simulink library "GenericINSLibrary"  (R2020b)
settings: Solver=VariableStepAuto  StartTime=0.0  StopTime=10.0  RelTol=1e-3
libraries: simulink x44
(part 5 of 6)

== matlab function GenericINSLibrary/Sensor Fusion/MATLAB Function ==
  data: time input; initialState input; valid output; initialStdDev input; reset input; sampletime input; IMU_Data input; IMU_StdDev input; IMU_PositionBody2Sensor input; IMU_DCMBody2Sensor input; P1_Data input; P1_StdDev input; P1_PositionBody2Sensor input; P2_Data input; P2_StdDev input; P2_PositionBody2Sensor input; P3_Data input; P3_StdDev input; P3_PositionBody2Sensor input; P4_Data input; P4_StdDev input; P4_PositionBody2Sensor input; P5_Data input; P5_StdDev input; P5_PositionBody2Sensor input; P6_Data input; P6_StdDev input; P6_PositionBody2Sensor input; V1_Data input; V1_StdDev input; V1_PositionBody2Sensor input; V1_DCMBody2Sensor input; V2_Data input; V2_StdDev input; V2_PositionBody2Sensor input; V2_DCMBody2Sensor input; V3_Data input; V3_StdDev input; V3_PositionBody2Sensor input; V3_DCMBody2Sensor input; V4_Data input; V4_StdDev input; V4_PositionBody2Sensor input; V4_DCMBody2Sensor input; O1_Data input; O1_StdDev input; O1_DCMBody2Sensor input; O2_Data input; O2_StdDev input; O2_DCMBody2Sensor input; O3_Data input; O3_StdDev input; O3_DCMBody2Sensor input; O4_Data input; O4_StdDev input; O4_DCMBody2Sensor input; SOG1_Data input; SOG1_StdDev input; SOG1_PositionBody2Sensor input; SOG2_Data input; SOG2_StdDev input; SOG2_PositionBody2Sensor input; SOG3_Data input; SOG3_StdDev input; SOG3_PositionBody2Sensor input; SOG4_Data input; SOG4_StdDev input; SOG4_PositionBody2Sensor input; SOG5_Data input; SOG5_StdDev input; SOG5_PositionBody2Sensor input; SOG6_Data input; SOG6_StdDev input; SOG6_PositionBody2Sensor input; numPredictions output; numUpdates output; positionLLA output; orientationQuaternionWXYZ output; orientationRollPitchYaw output; velocityNED output; velocityUVW output; velocityPQR output; courseOverGround output; speedOverGround output; angleOfAttack output; sideSlipAngle output; inertialSensorBias output; internalX output; internalS output
function [valid, numPredictions, numUpdates, positionLLA, orientationQuaternionWXYZ, orientationRollPitchYaw, velocityNED, velocityUVW, velocityPQR, courseOverGround, speedOverGround, angleOfAttack, sideSlipAngle, inertialSensorBias, internalX, internalS] = MultiSensorFusion(time, initialState, initialStdDev, reset, sampletime, IMU_Data, IMU_StdDev, IMU_PositionBody2Sensor, IMU_DCMBody2Sensor, P1_Data, P1_StdDev, P1_PositionBody2Sensor, P2_Data, P2_StdDev, P2_PositionBody2Sensor, P3_Data, P3_StdDev, P3_PositionBody2Sensor, P4_Data, P4_StdDev, P4_PositionBody2Sensor, P5_Data, P5_StdDev, P5_PositionBody2Sensor, P6_Data, P6_StdDev, P6_PositionBody2Sensor, V1_Data, V1_StdDev, V1_PositionBody2Sensor, V1_DCMBody2Sensor, V2_Data, V2_StdDev, V2_PositionBody2Sensor, V2_DCMBody2Sensor, V3_Data, V3_StdDev, V3_PositionBody2Sensor, V3_DCMBody2Sensor, V4_Data, V4_StdDev, V4_PositionBody2Sensor, V4_DCMBody2Sensor, O1_Data, O1_StdDev, O1_DCMBody2Sensor, O2_Data, O2_StdDev, O2_DCMBody2Sensor, O3_Data, O3_StdDev, O3_DCMBody2Sensor, O4_Data, O4_StdDev, O4_DCMBody2Sensor, SOG1_Data, SOG1_StdDev, SOG1_PositionBody2Sensor, SOG2_Data, SOG2_StdDev, SOG2_PositionBody2Sensor, SOG3_Data, SOG3_StdDev, SOG3_PositionBody2Sensor, SOG4_Data, SOG4_StdDev, SOG4_PositionBody2Sensor, SOG5_Data, SOG5_StdDev, SOG5_PositionBody2Sensor, SOG6_Data, SOG6_StdDev, SOG6_PositionBody2Sensor)
    %MultiSensorFusion Generated MATLAB function for a generic inertial navigation system (6 position measurements, 4 velocity measurements, 4 orientation measurements).
    % This function was automatically generated using the command GenericINS.SensorFusion.GenerateFunction('MultiSensorFusion', [3  3  3  3  3  3], [3  3  2  2], [3  3  1  1], 6).
    % 
    % PARAMETERS
    % time                       ... A scalar value indicating a monotonically increasing time in seconds.
    % initialState               ... 15-by-1 initial state vector to be used when the INS is reset. The elements are as follows:
    %                                 1: latitude     [rad]     Initial latitude of the position of the IMU.
    %                                 2: longitude    [rad]     Initial longitude of the position of the IMU.
    %                                 3: altitude     [m]       Initial altitude of the position of the IMU, positive upwards.
    %                                 4: velocityU    [m/s]     Initial body-fixed velocity in x-direction of the body-frame at the position of the IMU.
    %                                 5: velocityV    [m/s]     Initial body-fixed velocity in y-direction of the body-frame at the position of the IMU.
    %                                 6: velocityW    [m/s]     Initial body-fixed velocity in z-direction of the body-frame at the position of the IMU.
    %                                 7: roll         [rad]     Initial roll angle.
    %                                 8: pitch        [rad]     Initial pitch angle.
    %                                 9: yaw          [rad]     Initial yaw angle.
    %                                10: biasAccX     [m/(s*s)] Initial acceleration bias in x-direction of IMU sensor frame.
    %                                11: biasAccY     [m/(s*s)] Initial acceleration bias in y-direction of IMU sensor frame.
    %                                12: biasAccZ     [m/(s*s)] Initial acceleration bias in z-direction of IMU sensor frame.
    %                                13: biasGyrX     [rad/s]   Initial angular rate bias around x-axis of IMU sensor frame.
    %                                14: biasGyrY     [rad/s]   Initial angular rate bias around y-axis of IMU sensor frame.
    %                                15: biasGyrZ     [rad/s]   Initial angular rate bias around z-axis of IMU sensor frame.
    % initialStdDev              ... 15-by-1 standard deviation vector that represents the unvertainty of the initial state. It is better to use larger values than
    %                                too small values for the filter to converge. The elements are as follows:
    %                                 1: latitude     [rad]     Initial standard deviation for initial latitude.
    %                                 2: longitude    [rad]     Initial standard deviation for initial longitude.
    %                                 3: altitude     [m]       Initial standard deviation for initial altitude.
    %                                 4: velocityU    [m/s]     Initial standard deviation for initial body-fixed velocity in x-direction of the body-frame.
    %                                 5: velocityV    [m/s]     Initial standard deviation for initial body-fixed velocity in y-direction of the body-frame.
    %                                 6: velocityW    [m/s]     Initial standard deviation for initial body-fixed velocity in z-direction of the body-frame.
    %                                 7: orientationX           Initial standard deviation for x-component of orientation vector (axis-angle representation).
    %                                 8: orientationY           Initial standard deviation for y-component of orientation vector (axis-angle representation).
    %                                 9: orientationZ           Initial standard deviation for z-component of orientation vector (axis-angle representation).
    %                                10: biasAccX     [m/(s*s)] Initial standard deviation for acceleration bias in x-direction of IMU sensor frame.
    %                                11: biasAccY     [m/(s*s)] Initial standard deviation for acceleration bias in y-direction of IMU sensor frame.
    %                                12: biasAccZ     [m/(s*s)] Initial standard deviation for acceleration bias in z-direction of IMU sensor frame.
    %                                13: biasGyrX     [rad/s]   Initial standard deviation for angular rate bias around x-axis of IMU sensor frame.
    %                                14: biasGyrY     [rad/s]   Initial standard deviation for angular rate bias around y-axis of IMU sensor frame.
    %                                15: biasGyrZ     [rad/s]   Initial standard deviation for angular rate bias around z-axis of IMU sensor frame.
    % reset                      ... Greater than 0.0 if filter should be reset/reinitialized, 0.0 otherwise. During an initialization the initial state and initial standard deviations are used.
    % sampletime                 ... Discrete sampletime in seconds to be used for forward euler integration. Should be the elapsed time to the latest prediction.
    % IMU_Data                   ... The 7-by-1 vector representing the IMU data where the elements are as follows:
    %                                 1: trigger                Greater than 0.0 if new IMU data is available and should be used in a prediction step, 0.0 otherwise.
    %                                 2: accX         [m/(s*s)] Acceleration in x-direction of IMU sensor frame.
    %                                 3: accY         [m/(s*s)] Acceleration in y-direction of IMU sensor frame.
    %                                 4: accZ         [m/(s*s)] Acceleration in z-direction of IMU sensor frame.
    %                                 5: gyrX         [rad/s]   Angular rate around x-axis of IMU sensor frame.
    %                                 6: gyrY         [rad/s]   Angular rate around y-axis of IMU sensor frame.
    %                                 7: gyrZ         [rad/s]   Angular rate around z-axis of IMU sensor frame.
    % IMU_StdDev                 ... 12-by-1 vector representing the standard deviation for inertial measurements and inertial biases. The elements are as follows:
    %                                 1: accX         [m/(s*s)] Standard deviation for acceleration in x-direction of IMU sensor frame.
    %                                 2: accY         [m/(s*s)] Standard deviation for acceleration in y-direction of IMU sensor frame.
    %                                 3: accZ         [m/(s*s)] Standard deviation for acceleration in z-direction of IMU sensor frame.
    %                                 4: gyrX         [rad/s]   Standard deviation for angular rate around x-axis of IMU sensor frame.
    %                                 5: gyrY         [rad/s]   Standard deviation for angular rate around y-axis of IMU sensor frame.
    %                                 6: gyrZ         [rad/s]   Standard deviation for angular rate around z-axis of IMU sensor frame.
    %                                 7: biasAccX     [m/(s*s)] Standard deviation for acceleration bias in x-direction of IMU sensor frame.
    %                                 8: biasAccY     [m/(s*s)] Standard deviation for acceleration bias in y-direction of IMU sensor frame.
    %                                 9: biasAccZ     [m/(s*s)] Standard deviation for acceleration bias in z-direction of IMU sensor frame.
    %                                10: biasGyrX     [rad/s]   Standard deviation for angular rate bias around x-axis of IMU sensor frame.
    %                                11: biasGyrY     [rad/s]   Standard deviation for angular rate bias around y-axis of IMU sensor frame.
    %                                12: biasGyrZ     [rad/s]   Standard deviation for angular rate bias around z-axis of IMU sensor frame.
    % IMU_PositionBody2Sensor    ... Position of IMU sensor frame origin w.r.t. body frame origin in body frame coordinates (meters).
    % IMU_DCMBody2Sensor         ... Direction cosine matrix to rotate measurements from body frame to sensor frame.
    % P1_Data                    ... 4-by-1 vector representing the position measurements of position sensor 1. The elements are as follows:
    %                                 1: trigger                Greater than 0.0 if new measurement data is available and should be used in an update step, 0.0 otherwise.
    %                                 2: latitude     [rad]     The latitude measurement.
    %                                 3: longitude    [rad]     The longitude measurement.
    %                                 4: altitude     [m]       The altitude measurement.
    % P1_StdDev                  ... 3-by-1 vector representing the standard deviation for the position measurements of position sensor 1. The elements are as follows:
    %                                 1: stdNorth     [m]       Standard deviation in north direction.
    %                                 2: stdEast      [m]       Standard deviation in east direction.
    %                                 3: stdDown      [m]       Standard deviation in up/down-direction.
    % P1_PositionBody2Sensor     ... Position of position sensor 1 w.r.t. body frame origin in body frame coordinates (meters).
    % P2_Data                    ... 4-by-1 vector representing the position measurements of position sensor 2. The elements are as follows:
    %                                 1: trigger                Greater than 0.0 if new measurement data is available and should be used in an update step, 0.0 otherwise.
    %                                 2: latitude     [rad]     The latitude measurement.
    %                                 3: longitude    [rad]     The longitude measurement.
    %                                 4: altitude     [m]       The altitude measurement.
    % P2_StdDev                  ... 3-by-1 vector representing the standard deviation for the position measurements of position sensor 2. The elements are as follows:
    %                                 1: stdNorth     [m]       Standard deviation in north direction.
    %                                 2: stdEast      [m]       Standard deviation in east direction.
    %                                 3: stdDown      [m]       Standard deviation in up/down-direction.
    % P2_PositionBody2Sensor     ... Position of position sensor 2 w.r.t. body frame origin in body frame coordinates (meters).
    % P3_Data                    ... 4-by-1 vector representing the position measurements of position sensor 3. The elements are as follows:
    %                                 1: trigger                Greater than 0.0 if new measurement data is available and should be used in an update step, 0.0 otherwise.
    %                                 2: latitude     [rad]     The latitude measurement.
    %                                 3: longitude    [rad]     The longitude measurement.
    %                                 4: altitude     [m]       The altitude measurement.
    % P3_StdDev                  ... 3-by-1 vector representing the standard deviation for the position measurements of position sensor 3. The elements are as follows:
    %                                 1: stdNorth     [m]       Standard deviation in north direction.
    %                                 2: stdEast      [m]       Standard deviation in east direction.
    %                                 3: stdDown      [m]       Standard deviation in up/down-direction.
    % P3_PositionBody2Sensor     ... Position of position sensor 3 w.r.t. body frame origin in body frame coordinates (meters).
    % P4_Data                    ... 4-by-1 vector representing the position measurements of position sensor 4. The elements are as follows:
    %                                 1: trigger                Greater than 0.0 if new measurement data is available and should be used in an update step, 0.0 otherwise.
    %                                 2: latitude     [rad]     The latitude measurement.
    %                                 3: longitude    [rad]     The longitude measurement.
    %                                 4: altitude     [m]       The altitude measurement.
    % P4_StdDev                  ... 3-by-1 vector representing the standard deviation for the position measurements of position sensor 4. The elements are as follows:
    %                                 1: stdNorth     [m]       Standard deviation in north direction.
    %                                 2: stdEast      [m]       Standard deviation in east direction.
    %                                 3: stdDown      [m]       Standard deviation in up/down-direction.
    % P4_PositionBody2Sensor     ... Position of position sensor 4 w.r.t. body frame origin in body frame coordinates (meters).
    % P5_Data                    ... 4-by-1 vector representing the position measurements of position sensor 5. The elements are as follows:
    %                                 1: trigger                Greater than 0.0 if new measurement data is available and should be used in an update step, 0.0 otherwise.
    %                                 2: latitude     [rad]     The latitude measurement.
    %                                 3: longitude    [rad]     The longitude measurement.
    %                                 4: altitude     [m]       The altitude measurement.
    % P5_StdDev                  ... 3-by-1 vector representing the standard deviation for the position measurements of position sensor 5. The elements are as follows:
    %                                 1: stdNorth     [m]       Standard deviation in north direction.
    %                                 2: stdEast      [m]       Standard deviation in east direction.
    %                                 3: stdDown      [m]       Standard deviation in up/down-direction.
    % P5_PositionBody2Sensor     ... Position of position sensor 5 w.r.t. body frame origin in body frame coordinates (meters).
    % P6_Data                    ... 4-by-1 vector representing the position measurements of position sensor 6. The elements are as follows:
    %                                 1: trigger                Greater than 0.0 if new measurement data is available and should be used in an update step, 0.0 otherwise.
    %                                 2: latitude     [rad]     The latitude measurement.
    %                                 3: longitude    [rad]     The longitude measurement.
    %                                 4: altitude     [m]       The altitude measurement.
    % P6_StdDev                  ... 3-by-1 vector representing the standard deviation for the position measurements of position sensor 6. The elements are as follows:
    %                                 1: stdNorth     [m]       Standard deviation in north direction.
    %                                 2: stdEast      [m]       Standard deviation in east direction.
    %                                 3: stdDown      [m]       Standard deviation in up/down-direction.
    % P6_PositionBody2Sensor     ... Position of position sensor 6 w.r.t. body frame origin in body frame coordinates (meters).
    % V1_Data                    ... 4-by-1 vector representing the velocity measurements of velocity sensor 1. The elements are as follows:
    %                                 1: trigger                Greater than 0.0 if new measurement data is available and should be used in an update step, 0.0 otherwise.
    %                                 2: velocityX    [m/s]     The velocity measurement in x-direction of sensor frame.
    %                                 3: velocityY    [m/s]     The velocity measurement in y-direction of sensor frame.
    %                                 4: velocityZ    [m/s]     The velocity measurement in z-direction of sensor frame.
    % V1_StdDev                  ... 3-by-1 vector representing the standard deviation for the velocity measurements of velocity sensor 1. The elements are as follows:
    %                                 1: stdX         [m/s]     Standard deviation in x-direction.
    %                                 2: stdY         [m/s]     Standard deviation in y-direction.
    %                                 3: stdZ         [m/s]     Standard deviation in z-direction.
    % V1_PositionBody2Sensor     ... Position of velocity sensor 1 w.r.t. body frame origin in body frame coordinates (meters).
    % V1_DCMBody2Sensor          ... Direction cosine matrix to rotate vectors from body frame to sensor frame.
    % V2_Data                    ... 4-by-1 vector representing the velocity measurements of velocity sensor 2. The elements are as follows:
    %                                 1: trigger                Greater than 0.0 if new measurement data is available and should be used in an update step, 0.0 otherwise.
    %                                 2: velocityX    [m/s]     The velocity measurement in x-direction of sensor frame.
    %                                 3: velocityY    [m/s]     The velocity measurement in y-direction of sensor frame.
    %                                 4: velocityZ    [m/s]     The velocity measurement in z-direction of sensor frame.
    % V2_StdDev                  ... 3-by-1 vector representing the standard deviation for the velocity measurements of velocity sensor 2. The elements are as follows:
    %                                 1: stdX         [m/s]     Standard deviation in x-direction.
    %                                 2: stdY         [m/s]     Standard deviation in y-direction.
    %                                 3: stdZ         [m/s]     Standard deviation in z-direction.
    % V2_PositionBody2Sensor     ... Position of velocity sensor 2 w.r.t. body frame origin in body frame coordinates (meters).
    % V2_DCMBody2Sensor          ... Direction cosine matrix to rotate vectors from body frame to sensor frame.
    % V3_Data                    ... 3-by-1 vector representing the velocity measurements of velocity sensor 3. The elements are as follows:
    %                                 1: trigger                Greater than 0.0 if new measurement data is available and should be used in an update step, 0.0 otherwise.
    %                                 2: velocityX    [m/s]     The velocity measurement in x-direction of sensor frame.
    %                                 3: velocityY    [m/s]     The velocity measurement in y-direction of sensor frame.
    % V3_StdDev                  ... 2-by-1 vector representing the standard deviation for the velocity measurements of velocity sensor 3. The elements are as follows:
    %                                 1: stdX         [m/s]     Standard deviation in x-direction.
    %                                 2: stdY         [m/s]     Standard deviation in y-direction.
    % V3_PositionBody2Sensor     ... Position of velocity sensor 3 w.r.t. body frame origin in body frame coordinates (meters).
    % V3_DCMBody2Sensor          ... Direction cosine matrix to rotate vectors from body frame to sensor frame.
    % V4_Data                    ... 3-by-1 vector representing the velocity measurements of velocity sensor 4. The elements are as follows:
    %                                 1: trigger                Greater than 0.0 if new measurement data is available and should be used in an update step, 0.0 otherwise.
    %                                 2: velocityX    [m/s]     The velocity measurement in x-direction of sensor frame.
    %                                 3: velocityY    [m/s]     The velocity measurement in y-direction of sensor frame.
    % V4_StdDev                  ... 2-by-1 vector representing the standard deviation for the velocity measurements of velocity sensor 4. The elements are as follows:
    %                                 1: stdX         [m/s]     Standard deviation in x-direction.
    %                                 2: stdY         [m/s]     Standard deviation in y-direction.
    % V4_PositionBody2Sensor     ... Position of velocity sensor 4 w.r.t. body frame origin in body frame coordinates (meters).
    % V4_DCMBody2Sensor          ... Direction cosine matrix to rotate vectors from body frame to sensor frame.
    % O1_Data                    ... 4-by-1 vector representing the orientation measurements of orientation sensor 1. Note that orientation measurements must only be used for applications with small roll and pitch angles. The elements are as follows:
    %                                 1: trigger                Greater than 0.0 if new measurement data is available and should be used in an update step, 0.0 otherwise.
    %                                 2: roll         [rad]     The roll angle measurement (ZYX-convention).
    %                                 3: pitch        [rad]     The pitch angle measurement (ZYX-convention).
    %                                 4: yaw          [rad]     The yaw angle measurement (ZYX-convention).
    % O1_StdDev                  ... 3-by-1 vector representing the standard deviation for the orientation measurements of orientation sensor 1. The elements are as follows:
    %                                 1: stdRoll      [rad]     Standard deviation for roll angle.
    %                                 2: stdPitch     [rad]     Standard deviation for pitch angle.
    %                                 3: stdYaw       [rad]     Standard deviation for yaw angle.
    % O1_DCMBody2Sensor          ... Direction cosine matrix to rotate vectors from body frame to sensor frame.
    % O2_Data                    ... 4-by-1 vector representing the orientation measurements of orientation sensor 2. Note that orientation measurements must only be used for applications with small roll and pitch angles. The elements are as follows:
    %                                 1: trigger                Greater than 0.0 if new measurement data is available and should be used in an update step, 0.0 otherwise.
    %                                 2: roll         [rad]     The roll angle measurement (ZYX-convention).
    %                                 3: pitch        [rad]     The pitch angle measurement (ZYX-convention).
    %                                 4: yaw          [rad]     The yaw angle measurement (ZYX-convention).
    % O2_StdDev                  ... 3-by-1 vector representing the standard deviation for the orientation measurements of orientation sensor 2. The elements are as follows:
    %                                 1: stdRoll      [rad]     Standard deviation for roll angle.
    %                                 2: stdPitch     [rad]     Standard deviation for pitch angle.
    %                                 3: stdYaw       [rad]     Standard deviation for yaw angle.
    % O2_DCMBody2Sensor          ... Direction cosine matrix to rotate vectors from body frame to sensor frame.
    % O3_Data                    ... 2-by-1 vector representing the orientation measurements of orientation sensor 3. Note that orientation measurements must only be used for applications with small roll and pitch angles. The elements are as follows:
    %                                 1: trigger                Greater than 0.0 if new measurement data is available and should be used in an update step, 0.0 otherwise.
    %                                 2: yaw          [rad]     The yaw angle measurement (ZYX-convention).
    % O3_StdDev                  ... 1-by-1 vector representing the standard deviation for the orientation measurements of orientation sensor 3. The elements are as follows:
    %                                 1: stdYaw       [rad]     Standard deviation for yaw angle.
    % O3_DCMBody2Sensor          ... Direction cosine matrix to rotate vectors from body frame to sensor frame.
    % O4_Data                    ... 2-by-1 vector representing the orientation measurements of orientation sensor 4. Note that orientation measurements must only be used for applications with small roll and pitch angles. The elements are as follows:
    %                                 1: trigger                Greater than 0.0 if new measurement data is available and should be used in an update step, 0.0 otherwise.
    %                                 2: yaw          [rad]     The yaw angle measurement (ZYX-convention).
    % O4_StdDev                  ... 1-by-1 vector representing the standard deviation for the orientation measurements of orientation sensor 4. The elements are as follows:
    %                                 1: stdYaw       [rad]     Standard deviation for yaw angle.
    % O4_DCMBody2Sensor          ... Direction cosine matrix to rotate vectors from body frame to sensor frame.
    % SOG1_Data                  ... 2-by-1 vector representing the speed-over-ground measurements of SOG sensor 1. The elements are as follows:
    %                                 1: trigger                Greater than 0.0 if new measurement data is available and should be used in an update step, 0.0 otherwise.
    %                                 2: speedOverGround [m/s]     The velocity measurement in z-direction of sensor frame.
    % SOG1_StdDev                ... Scalar value representing the standard deviation for the speed-over-ground measurement of SOG sensor 1 in [m/s].
    % SOG1_PositionBody2Sensor   ... Position of SOG sensor 1 w.r.t. body frame origin in body frame coordinates (meters).
    % SOG2_Data                  ... 2-by-1 vector representing the speed-over-ground measurements of SOG sensor 2. The elements are as follows:
    %                                 1: trigger                Greater than 0.0 if new measurement data is available and should be used in an update step, 0.0 otherwise.
    %                                 2: speedOverGround [m/s]     The velocity measurement in z-direction of sensor frame.
    % SOG2_StdDev                ... Scalar value representing the standard deviation for the speed-over-ground measurement of SOG sensor 2 in [m/s].
    % SOG2_PositionBody2Sensor   ... Position of SOG sensor 2 w.r.t. body frame origin in body frame coordinates (meters).
    % SOG3_Data                  ... 2-by-1 vector representing the speed-over-ground measurements of SOG sensor 3. The elements are as follows:
    %                                 1: trigger                Greater than 0.0 if new measurement data is available and should be used in an update step, 0.0 otherwise.
    %                                 2: speedOverGround [m/s]     The velocity measurement in z-direction of sensor frame.
    % SOG3_StdDev                ... Scalar value representing the standard deviation for the speed-over-ground measurement of SOG sensor 3 in [m/s].
    % SOG3_PositionBody2Sensor   ... Position of SOG sensor 3 w.r.t. body frame origin in body frame coordinates (meters).
    % SOG4_Data                  ... 2-by-1 vector representing the speed-over-ground measurements of SOG sensor 4. The elements are as follows:
    %                                 1: trigger                Greater than 0.0 if new measurement data is available and should be used in an update step, 0.0 otherwise.
    %                                 2: speedOverGround [m/s]     The velocity measurement in z-direction of sensor frame.
    % SOG4_StdDev                ... Scalar value representing the standard deviation for the speed-over-ground measurement of SOG sensor 4 in [m/s].
    % SOG4_PositionBody2Sensor   ... Position of SOG sensor 4 w.r.t. body frame origin in body frame coordinates (meters).
    % SOG5_Data                  ... 2-by-1 vector representing the speed-over-ground measurements of SOG sensor 5. The elements are as follows:
    %                                 1: trigger                Greater than 0.0 if new measurement data is available and should be used in an update step, 0.0 otherwise.
    %                                 2: speedOverGround [m/s]     The velocity measurement in z-direction of sensor frame.
    % SOG5_StdDev                ... Scalar value representing the standard deviation for the speed-over-ground measurement of SOG sensor 5 in [m/s].
    % SOG5_PositionBody2Sensor   ... Position of SOG sensor 5 w.r.t. body frame origin in body frame coordinates (meters).
    % SOG6_Data                  ... 2-by-1 vector representing the speed-over-ground measurements of SOG sensor 6. The elements are as follows:
    %                                 1: trigger                Greater than 0.0 if new measurement data is available and should be used in an update step, 0.0 otherwise.
    %                                 2: speedOverGround [m/s]     The velocity measurement in z-direction of sensor frame.
    % SOG6_StdDev                ... Scalar value representing the standard deviation for the speed-over-ground measurement of SOG sensor 6 in [m/s].
    % SOG6_PositionBody2Sensor   ... Position of SOG sensor 6 w.r.t. body frame origin in body frame coordinates (meters).
    % 
    % RETURN
    % valid                      ... A scalar boolean that indicates whether the motion state is valid or not. It is valid if the INS was initialized.
    % numPredictions             ... An integer indicating the number of prediction steps that have been calculated (either 0 or 1).
    % numUpdates                 ... An integer indicating the number of update steps that have been calculated.
    % positionLLA                ... Geographic position of the body frame, [lat (rad); lon (rad); alt (m, positive upwards)].
    % orientationQuaternionWXYZ  ... Unit quaternion describing a rotation from body frame to navigation frame, [qw; qx; qy; qz], where qw indicates the scalar part of the quaternion.
    % orientationRollPitchYaw    ... Euler angles according to the ZYX-convention.
    % velocityNED                ... Translational velocity [m/s] of the body frame given in navigation frame coordinates, excluding earth rotation and transport rate.
    % velocityUVW                ... Translational velocity [m/s] of the body frame given in body frame coordinates, excluding earth rotation and transport rate.
    % velocityPQR                ... Rotational velocity [rad/s] of the body frame with respect to the navigation frame, excluding earth rotation and transport rate.
    % courseOverGround           ... Course over ground angle in radians.
    % speedOverGround            ... Speed over ground in meters per second.
    % angleOfAttack              ... Angle of attack in radians.
    % sideSlipAngle              ... Side slip angle in radians.
    % inertialSensorBias         ... Inertial sensor bias [accX (m/s^2); accY (m/s^2); accZ (m/s^2); gyrX (rad/s); gyrY (rad/s); gyrZ (rad/s)].
    % internalX                  ... 16-by-1 state vector representing the internal motion state with respect to the IMU. Elements are as follows:
    %                            ...  1: Latitude in radians.
    %                            ...  2: Longitude in radians.
    %                            ...  3: Altitude in meters (positive upwards).
    %                            ...  4: North velocity in meters per second.
    %                            ...  5: East velocity in meters per second.
    %                            ...  6: Down velocity in meters per second.
    %                            ...  7: Scalar part of unit quaternion.
    %                            ...  8: First element of vector part of unit quaternion.
    %                            ...  9: Second element of vector part of unit quaternion.
    %                            ... 10: Third element of vector part of unit quaternion.
    %                            ... 11: Accelerometer bias (x) in m/s^2.
    %                            ... 12: Accelerometer bias (y) in m/s^2.
    %                            ... 13: Accelerometer bias (z) in m/s^2.
    %                            ... 14: Gyroscope bias (x) in rad/s.
    %                            ... 15: Gyroscope bias (x) in rad/s.
    %                            ... 16: Gyroscope bias (x) in rad/s.
    % internalS                  ... 15-by-15 matrix representing the internal square root of the state covariance matrix. This matrix relates to the internalX state. Note that the uncertainty of the quaternion (4D) is represented by an orientation vector (3D).
    assert(isscalar(time) && (15 == size(initialState,1)) && (1 == size(initialState,2)) && (15 == size(initialStdDev,1)) && (1 == size(initialStdDev,2)) && isscalar(reset) && isscalar(sampletime) && (7 == size(IMU_Data,1)) && (1 == size(IMU_Data,2)) && (3 == size(IMU_PositionBody2Sensor,1)) && (1 == size(IMU_PositionBody2Sensor,2)) && (3 == size(IMU_DCMBody2Sensor,1)) && (3 == size(IMU_DCMBody2Sensor,2)));
    persistent prevTime; if(isempty(prevTime)), prevTime = time; end
    persistent ins; if(isempty(ins)), ins = GenericINS.SensorFusion(); end
    persistent imuStdDevBuffer; if(isempty(imuStdDevBuffer)), imuStdDevBuffer = IMU_StdDev; end

    assert((4 == size(P1_Data,1)) && (1 == size(P1_Data,2)) && (3 == size(P1_StdDev,1)) && (1 == size(P1_StdDev,2)) && (3 == size(P1_PositionBody2Sensor,1)) && (1 == size(P1_PositionBody2Sensor,2)));
    persistent P1_Buffer; if(isempty(P1_Buffer) || (P1_Data(1) > 0.0)), P1_Buffer = P1_Data; end
    assert((4 == size(P2_Data,1)) && (1 == size(P2_Data,2)) && (3 == size(P2_StdDev,1)) && (1 == size(P2_StdDev,2)) && (3 == size(P2_PositionBody2Sensor,1)) && (1 == size(P2_PositionBody2Sensor,2)));
    persistent P2_Buffer; if(isempty(P2_Buffer) || (P2_Data(1) > 0.0)), P2_Buffer = P2_Data; end
    assert((4 == size(P3_Data,1)) && (1 == size(P3_Data,2)) && (3 == size(P3_StdDev,1)) && (1 == size(P3_StdDev,2)) && (3 == size(P3_PositionBody2Sensor,1)) && (1 == size(P3_PositionBody2Sensor,2)));
    persistent P3_Buffer; if(isempty(P3_Buffer) || (P3_Data(1) > 0.0)), P3_Buffer = P3_Data; end
    assert((4 == size(P4_Data,1)) && (1 == size(P4_Data,2)) && (3 == size(P4_StdDev,1)) && (1 == size(P4_StdDev,2)) && (3 == size(P4_PositionBody2Sensor,1)) && (1 == size(P4_PositionBody2Sensor,2)));
    persistent P4_Buffer; if(isempty(P4_Buffer) || (P4_Data(1) > 0.0)), P4_Buffer = P4_Data; end
    assert((4 == size(P5_Data,1)) && (1 == size(P5_Data,2)) && (3 == size(P5_StdDev,1)) && (1 == size(P5_StdDev,2)) && (3 == size(P5_PositionBody2Sensor,1)) && (1 == size(P5_PositionBody2Sensor,2)));
    persistent P5_Buffer; if(isempty(P5_Buffer) || (P5_Data(1) > 0.0)), P5_Buffer = P5_Data; end
    assert((4 == size(P6_Data,1)) && (1 == size(P6_Data,2)) && (3 == size(P6_StdDev,1)) && (1 == size(P6_StdDev,2)) && (3 == size(P6_PositionBody2Sensor,1)) && (1 == size(P6_PositionBody2Sensor,2)));
    persistent P6_Buffer; if(isempty(P6_Buffer) || (P6_Data(1) > 0.0)), P6_Buffer = P6_Data; end
    assert((4 == size(V1_Data,1)) && (1 == size(V1_Data,2)) && (3 == size(V1_StdDev,1)) && (1 == size(V1_StdDev,2)) && (3 == size(V1_PositionBody2Sensor,1)) && (1 == size(V1_PositionBody2Sensor,2)) && (3 == size(V1_DCMBody2Sensor,1)) && (3 == size(V1_DCMBody2Sensor,2)));
    persistent V1_Buffer; if(isempty(V1_Buffer) || (V1_Data(1) > 0.0)), V1_Buffer = V1_Data; end
    assert((4 == size(V2_Data,1)) && (1 == size(V2_Data,2)) && (3 == size(V2_StdDev,1)) && (1 == size(V2_StdDev,2)) && (3 == size(V2_PositionBody2Sensor,1)) && (1 == size(V2_PositionBody2Sensor,2)) && (3 == size(V2_DCMBody2Sensor,1)) && (3 == size(V2_DCMBody2Sensor,2)));
    persistent V2_Buffer; if(isempty(V2_Buffer) || (V2_Data(1) > 0.0)), V2_Buffer = V2_Data; end
    assert((3 == size(V3_Data,1)) && (1 == size(V3_Data,2)) && (2 == size(V3_StdDev,1)) && (1 == size(V3_StdDev,2)) && (3 == size(V3_PositionBody2Sensor,1)) && (1 == size(V3_PositionBody2Sensor,2)) && (3 == size(V3_DCMBody2Sensor,1)) && (3 == size(V3_DCMBody2Sensor,2)));
    persistent V3_Buffer; if(isempty(V3_Buffer) || (V3_Data(1) > 0.0)), V3_Buffer = V3_Data; end
    assert((3 == size(V4_Data,1)) && (1 == size(V4_Data,2)) && (2 == size(V4_StdDev,1)) && (1 == size(V4_StdDev,2)) && (3 == size(V4_PositionBody2Sensor,1)) && (1 == size(V4_PositionBody2Sensor,2)) && (3 == size(V4_DCMBody2Sensor,1)) && (3 == size(V4_DCMBody2Sensor,2)));
    persistent V4_Buffer; if(isempty(V4_Buffer) || (V4_Data(1) > 0.0)), V4_Buffer = V4_Data; end
    assert((4 == size(O1_Data,1)) && (1 == size(O1_Data,2)) && (3 == size(O1_StdDev,1)) && (1 == size(O1_StdDev,2)) && (3 == size(O1_DCMBody2Sensor,1)) && (3 == size(O1_DCMBody2Sensor,2)));
    persistent O1_Buffer; if(isempty(O1_Buffer) || (O1_Data(1) > 0.0)), O1_Buffer = O1_Data; end
    assert((4 == size(O2_Data,1)) && (1 == size(O2_Data,2)) && (3 == size(O2_StdDev,1)) && (1 == size(O2_StdDev,2)) && (3 == size(O2_DCMBody2Sensor,1)) && (3 == size(O2_DCMBody2Sensor,2)));
    persistent O2_Buffer; if(isempty(O2_Buffer) || (O2_Data(1) > 0.0)), O2_Buffer = O2_Data; end
    assert((2 == size(O3_Data,1)) && (1 == size(O3_Data,2)) && (1 == size(O3_StdDev,1)) && (1 == size(O3_StdDev,2)) && (3 == size(O3_DCMBody2Sensor,1)) && (3 == size(O3_DCMBody2Sensor,2)));
    persistent O3_Buffer; if(isempty(O3_Buffer) || (O3_Data(1) > 0.0)), O3_Buffer = O3_Data; end
    assert((2 == size(O4_Data,1)) && (1 == size(O4_Data,2)) && (1 == size(O4_StdDev,1)) && (1 == size(O4_StdDev,2)) && (3 == size(O4_DCMBody2Sensor,1)) && (3 == size(O4_DCMBody2Sensor,2)));
    persistent O4_Buffer; if(isempty(O4_Buffer) || (O4_Data(1) > 0.0)), O4_Buffer = O4_Data; end
    assert((2 == size(SOG1_Data,1)) && (1 == size(SOG1_Data,2)) && (1 == size(SOG1_StdDev,1)) && (1 == size(SOG1_StdDev,2)) && (3 == size(SOG1_PositionBody2Sensor,1)) && (1 == size(SOG1_PositionBody2Sensor,2)));
    persistent SOG1_Buffer; if(isempty(SOG1_Buffer) || (SOG1_Data(1) > 0.0)), SOG1_Buffer = SOG1_Data; end
    assert((2 == size(SOG2_Data,1)) && (1 == size(SOG2_Data,2)) && (1 == size(SOG2_StdDev,1)) && (1 == size(SOG2_StdDev,2)) && (3 == size(SOG2_PositionBody2Sensor,1)) && (1 == size(SOG2_PositionBody2Sensor,2)));
    persistent SOG2_Buffer; if(isempty(SOG2_Buffer) || (SOG2_Data(1) > 0.0)), SOG2_Buffer = SOG2_Data; end
    assert((2 == size(SOG3_Data,1)) && (1 == size(SOG3_Data,2)) && (1 == size(SOG3_StdDev,1)) && (1 == size(SOG3_StdDev,2)) && (3 == size(SOG3_PositionBody2Sensor,1)) && (1 == size(SOG3_PositionBody2Sensor,2)));
    persistent SOG3_Buffer; if(isempty(SOG3_Buffer) || (SOG3_Data(1) > 0.0)), SOG3_Buffer = SOG3_Data; end
    assert((2 == size(SOG4_Data,1)) && (1 == size(SOG4_Data,2)) && (1 == size(SOG4_StdDev,1)) && (1 == size(SOG4_StdDev,2)) && (3 == size(SOG4_PositionBody2Sensor,1)) && (1 == size(SOG4_PositionBody2Sensor,2)));
    persistent SOG4_Buffer; if(isempty(SOG4_Buffer) || (SOG4_Data(1) > 0.0)), SOG4_Buffer = SOG4_Data; end
    assert((2 == size(SOG5_Data,1)) && (1 == size(SOG5_Data,2)) && (1 == size(SOG5_StdDev,1)) && (1 == size(SOG5_StdDev,2)) && (3 == size(SOG5_PositionBody2Sensor,1)) && (1 == size(SOG5_PositionBody2Sensor,2)));
    persistent SOG5_Buffer; if(isempty(SOG5_Buffer) || (SOG5_Data(1) > 0.0)), SOG5_Buffer = SOG5_Data; end
    assert((2 == size(SOG6_Data,1)) && (1 == size(SOG6_Data,2)) && (1 == size(SOG6_StdDev,1)) && (1 == size(SOG6_StdDev,2)) && (3 == size(SOG6_PositionBody2Sensor,1)) && (1 == size(SOG6_PositionBody2Sensor,2)));
    persistent SOG6_Buffer; if(isempty(SOG6_Buffer) || (SOG6_Data(1) > 0.0)), SOG6_Buffer = SOG6_Data; end

    imuStdDevChanged = (sum(abs(imuStdDevBuffer - IMU_StdDev) > 100*eps) > 0.0);
    eventReset = (reset > 0.0);
    if(eventReset)
        ins.Initialize(initialState(1:3), initialState(4:6), initialState(7:9), initialState(10:12), initialState(13:15), initialStdDev(1:3), initialStdDev(4:6), initialStdDev(7:9), initialStdDev(10:12), initialStdDev(13:15), IMU_StdDev(1:3), IMU_StdDev(4:6), IMU_StdDev(7:9), IMU_StdDev(10:12));
    elseif(imuStdDevChanged)
        ins.ResetInertialStandardDeviation(IMU_StdDev(1:3), IMU_StdDev(4:6), IMU_StdDev(7:9), IMU_StdDev(10:12));
    end
    imuStdDevBuffer = IMU_StdDev;
    numPredictions = int32(0);
    numUpdates = int32(0);
    if((IMU_Data(1) > 0.0) && ~eventReset)
        prevTime = time;

        % Motion prediction
        numPredictions = int32(1);
        ins.Predict(IMU_Data(2:7), sampletime, IMU_DCMBody2Sensor, IMU_PositionBody2Sensor);

        % Sensor updates
        if(P1_Buffer(1) > 0.0), numUpdates = numUpdates + int32(1); P1_Buffer(1) = 0.0; ins.UpdatePosition3D(P1_Buffer(2:end), P1_StdDev, P1_PositionBody2Sensor); end
        if(P2_Buffer(1) > 0.0), numUpdates = numUpdates + int32(1); P2_Buffer(1) = 0.0; ins.UpdatePosition3D(P2_Buffer(2:end), P2_StdDev, P2_PositionBody2Sensor); end
        if(P3_Buffer(1) > 0.0), numUpdates = numUpdates + int32(1); P3_Buffer(1) = 0.0; ins.UpdatePosition3D(P3_Buffer(2:end), P3_StdDev, P3_PositionBody2Sensor); end
        if(P4_Buffer(1) > 0.0), numUpdates = numUpdates + int32(1); P4_Buffer(1) = 0.0; ins.UpdatePosition3D(P4_Buffer(2:end), P4_StdDev, P4_PositionBody2Sensor); end
        if(P5_Buffer(1) > 0.0), numUpdates = numUpdates + int32(1); P5_Buffer(1) = 0.0; ins.UpdatePosition3D(P5_Buffer(2:end), P5_StdDev, P5_PositionBody2Sensor); end
        if(P6_Buffer(1) > 0.0), numUpdates = numUpdates + int32(1); P6_Buffer(1) = 0.0; ins.UpdatePosition3D(P6_Buffer(2:end), P6_StdDev, P6_PositionBody2Sensor); end
        if(V1_Buffer(1) > 0.0), numUpdates = numUpdates + int32(1); V1_Buffer(1) = 0.0; ins.UpdateVelocity3D(V1_Buffer(2:end), V1_StdDev, V1_PositionBody2Sensor, V1_DCMBody2Sensor); end
        if(V2_Buffer(1) > 0.0), numUpdates = numUpdates + int32(1); V2_Buffer(1) = 0.0; ins.UpdateVelocity3D(V2_Buffer(2:end), V2_StdDev, V2_PositionBody2Sensor, V2_DCMBody2Sensor); end
        if(V3_Buffer(1) > 0.0), numUpdates = numUpdates + int32(1); V3_Buffer(1) = 0.0; ins.UpdateVelocity2D(V3_Buffer(2:end), V3_StdDev, V3_PositionBody2Sensor, V3_DCMBody2Sensor); end
        if(V4_Buffer(1) > 0.0), numUpdates = numUpdates + int32(1); V4_Buffer(1) = 0.0; ins.UpdateVelocity2D(V4_Buffer(2:end), V4_StdDev, V4_PositionBody2Sensor, V4_DCMBody2Sensor); end
        if(O1_Buffer(1) > 0.0), numUpdates = numUpdates + int32(1); O1_Buffer(1) = 0.0; ins.UpdateOrientation3D(O1_Buffer(2:end), O1_StdDev, O1_DCMBody2Sensor); end
        if(O2_Buffer(1) > 0.0), numUpdates = numUpdates + int32(1); O2_Buffer(1) = 0.0; ins.UpdateOrientation3D(O2_Buffer(2:end), O2_StdDev, O2_DCMBody2Sensor); end
        if(O3_Buffer(1) > 0.0), numUpdates = numUpdates + int32(1); O3_Buffer(1) = 0.0; ins.UpdateOrientation1D(O3_Buffer(2:end), O3_StdDev, O3_DCMBody2Sensor); end
        if(O4_Buffer(1) > 0.0), numUpdates = numUpdates + int32(1); O4_Buffer(1) = 0.0; ins.UpdateOrientation1D(O4_Buffer(2:end), O4_StdDev, O4_DCMBody2Sensor); end
        if(SOG1_Buffer(1) > 0.0), numUpdates = numUpdates + int32(1); SOG1_Buffer(1) = 0.0; ins.UpdateSOG(SOG1_Buffer(2:end), SOG1_StdDev, SOG1_PositionBody2Sensor); end
        if(SOG2_Buffer(1) > 0.0), numUpdates = numUpdates + int32(1); SOG2_Buffer(1) = 0.0; ins.UpdateSOG(SOG2_Buffer(2:end), SOG2_StdDev, SOG2_PositionBody2Sensor); end
        if(SOG3_Buffer(1) > 0.0), numUpdates = numUpdates + int32(1); SOG3_Buffer(1) = 0.0; ins.UpdateSOG(SOG3_Buffer(2:end), SOG3_StdDev, SOG3_PositionBody2Sensor); end
        if(SOG4_Buffer(1) > 0.0), numUpdates = numUpdates + int32(1); SOG4_Buffer(1) = 0.0; ins.UpdateSOG(SOG4_Buffer(2:end), SOG4_StdDev, SOG4_PositionBody2Sensor); end
        if(SOG5_Buffer(1) > 0.0), numUpdates = numUpdates + int32(1); SOG5_Buffer(1) = 0.0; ins.UpdateSOG(SOG5_Buffer(2:end), SOG5_StdDev, SOG5_PositionBody2Sensor); end
        if(SOG6_Buffer(1) > 0.0), numUpdates = numUpdates + int32(1); SOG6_Buffer(1) = 0.0; ins.UpdateSOG(SOG6_Buffer(2:end), SOG6_StdDev, SOG6_PositionBody2Sensor); end
    end

    % Check for timeout
    if((time - prevTime) > 0.2)
        ins.MakeInvalid();
    end

    % Set output values
    [valid, positionLLA, orientationQuaternionWXYZ, orientationRollPitchYaw, velocityNED, velocityUVW, velocityPQR, courseOverGround, speedOverGround, angleOfAttack, sideSlipAngle, inertialSensorBias] = ins.GetMotionState();
    [internalX, internalS] = ins.GetInternalState();
    internalX = reshape(internalX, [16 1]);
    internalS = reshape(internalS, [15 15]);
end
